simulink model "etherCATmdl"  (R2022a)
settings: Solver=FixedStepDiscrete  StartTime=0.0  StopTime=inf  FixedStep=0.001  RelTol=1e-3
PreLoadFcn:
  | Ts_IO133 = 0.001;
  | Ts_IO750 = 0.001;
InitFcn:
  | Ts_IO133 = 0.001
StopFcn:
  | if isfile(['sdi_view_',bdroot,'.mldatx'])
  |  Simulink.sdi.clearPreferences();
  |  Simulink.sdi.view();
  |  pause(3);
  |  Simulink.sdi.loadView(['sdi_view_',bdroot,]);
  | end
undefined symbols (not defined in the file or in its folder): AUS0, AUS1, C, CAN, FD, padding, Statuswort, Steuerwort
libraries: speedgoatlib_IO750 x12, speedgoatlib_IO602 x9, slrealtimeutilitieslib x8, slrealtimeloglib x6, speedgoatlib_IO133 x5, canfdmsglib x4, canmsglib x4, etargetslib x2, slrealtimeptplib x2, speedgoatlib_interrupt x1, simulink x1
settings Model: SimulationMode=external  ExtModeEnableFloating=off  Creator=sandro.reichenbach  LastModifiedBy=muhammet.cingoez
settings SolverCC: ConcurrentTasks=on  PositivePriorityOrder=on  AutoInsertRateTranBlk=on
settings DataIOCC: LimitDataPoints=on  SaveFormat=StructureWithTime
settings OptimizationCC: BlockReduction=off  OptimizeBlockIOStorage=off
settings DebuggingCC: TasksWithSamePriorityMsg=none
settings HardwareCC: ProdBitPerLong=64  ProdLongLongMode=on  ProdHWDeviceType=Intel->x86-64 (Linux 64)
settings RTWCC: Description=Simulink Real-Time  SystemTargetFile=slrealtime.tlc  TemplateMakefile=slrealtime_default_tmf  PostCodeGenCommand=sg.model.build.makeCfg(bdroot, buildInfo);  RTWVerbose=off  Toolchain=Simulink Real-Time Toolchain  BuildConfiguration=Faster Runs  CodeExecutionProfiling=on  TargetLang=C++  DLArmComputeVersion=19.05

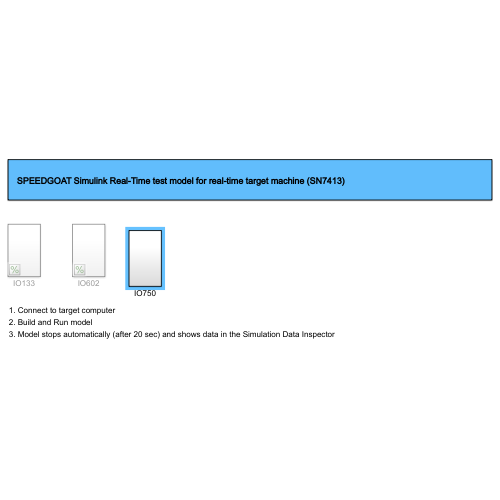
[thumbnail: Simulink's stored preview of the top-level diagram]
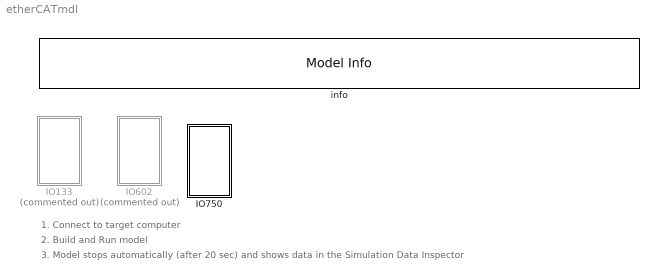
== system etherCATmdl ==
  note: 1. Connect to target computer
  note: 2. Build and Run model
  note: 3. Model stops automatically (after 20 sec) and shows data in the Simulation Data Inspector
  IO133 : Subsystem  Commented=on
  IO602 : Subsystem  Commented=on
  IO750 : Subsystem
  info : simulink/Model-Wide Utilities/Model Info  Frame=on  DisplayStringWithTags=SPEEDGOAT Simulink Real-Time test model for real-time target machine (SN7413)  HorizontalTextAlignment=Left  LeftAlignmentValue=0.02

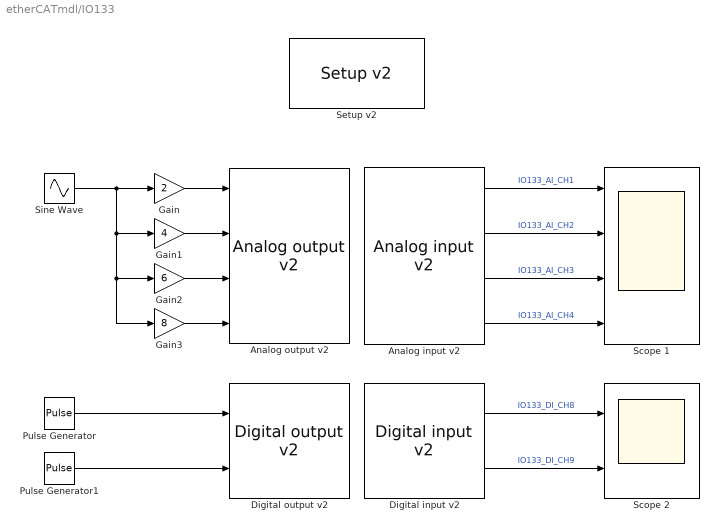
== system etherCATmdl/IO133 ==
  "Analog input v2 " : speedgoatlib_IO133/Analog input v2   parModuleId=1  parSampleTime=Ts_IO133  parPciSlot=-1  parAdcChannels=[1 2 3 4]  parAdcVoltageRange=[2 2]  parAdcOversamplRate=[1 1]  parAdcContSampling=0  parAdcDmaEnable=0  parAdcActiveDmaDevices=[1 1]  parAdcFrameSize=100
      settings: SourceProductName=Simulink Real-Time: Speedgoat I/O Driver Library
  "Analog output v2 " : speedgoatlib_IO133/Analog output v2   parModuleId=1  parSampleTime=Ts_IO133  parPciSlot=-1  parDacChannels=[1 2 3 4]  parDacVoltageRange=[4 4 6 6 5 5 5 5]  parDacInitValues=[0 0 0 0]  parDacReset=[1 1 1 1]  parDacSyncOut=1  parDacDmaEnable=0  parDacActiveDmaDevices=[1 1]  parDacDmaLatency=2  parDacFrameSize=100
      settings: SourceProductName=Simulink Real-Time: Speedgoat I/O Driver Library
  "Digital input v2 " : speedgoatlib_IO133/Digital input v2   parModuleId=1  parSampleTime=Ts_IO133  parPciSlot=-1  parDiChannels=[8 9]
      settings: SourceProductName=Simulink Real-Time: Speedgoat I/O Driver Library
  "Digital output v2 " : speedgoatlib_IO133/Digital output v2   parModuleId=1  parSampleTime=Ts_IO133  parPciSlot=-1  parDoChannels=[1 2]  parDoInitValues=[0 0]  parDoReset=[1 1]
      settings: SourceProductName=Simulink Real-Time: Speedgoat I/O Driver Library
  Gain : Gain  Gain=2
  Gain1 : Gain  Gain=4
  Gain2 : Gain  Gain=6
  Gain3 : Gain  Gain=8
  Pulse Generator : DiscretePulseGenerator  Period=20  PulseWidth=5  SampleTime=-1
  Pulse Generator1 : DiscretePulseGenerator  Period=20  PulseWidth=10  SampleTime=-1
  Scope 1 : Scope  NumInputPorts=4
  Scope 2 : Scope  NumInputPorts=2
  "Setup v2 " : speedgoatlib_IO133/Setup v2   parPciSlot=-1  parModuleId=1  parInterModuleSync=None  parConvClockBaseRate=20MHz  parConvClock1Divider=20000  parConvClock2Divider=20000  parFrameTriggerEnable=off  parFrameTriggerDivider=10  parConvClock1BaseRate=1  parConvClock2BaseRate=1  parFrameTriggerClock=1  parAdcChannels=1:4  parAdcRange1=+-10V  parAdcRange2=+-10V  parAdcVoltageRange=[2 2]  parAdcOversampling1=None  parAdcOversampling2=None  parAdcOversamplRate=[1 1]  parAdcAutoCorrection=on  parAdcContSampling=off  parAdcDmaEnable=off  parAdcDmaClock=Clock 1  parAdcFrameSize_=100  parAdcSampleTime_=-1  parAdcActiveDmaDevices=[1 1]  parAdcFrameTriggerEnable=0  parAdcFrameSize=100  parAdcSampleTime=0.1  parDacChannels=1:4  parDacInitValues=0  parDacReset=1  parDacRange1=+-5V  parDacRange2=+-5V  parDacRange3=+-10.8V  parDacRange4=+-10.8V  parDacRange5=+-10V  parDacRange6=+-10V  parDacRange7=+-10V  parDacRange8=+-10V  parDacVoltageRange=[4 4 6 6 5 5 5 5]  parDacAutoCorrection=on  parDacSyncOut=on  parDacDmaEnable=off  parDacDmaLatency=Until next frame  parDacDmaClock=Clock 1  parDacFrameSize_=100  parDacSampleTime_=-1  parDacActiveDmaDevices=[1 1]  parDacFrameTriggerEnable=0  parDacFrameSize=100  parDacSampleTime=0.1  parDoChannels=1:2  parDoInitValues=0  parDoReset=1  parDiChannels=8:9  parDiDebounceEnable=off  parDiDebounceTime=0  parDiDebounceValue=0  parDioPullRefFront=Pull-up 3.3V  parDioPullRefRear=Floating
      settings: SourceProductName=Simulink Real-Time: Speedgoat I/O Driver Library
  Sine Wave : Sin  Frequency=50  SampleTime=0
  wires:
  Pulse Generator/1 -> "Digital output v2 "/1
  Gain1/1 -> "Analog output v2 "/2
  Gain/1 -> "Analog output v2 "/1
  Gain3/1 -> "Analog output v2 "/4
  Gain2/1 -> "Analog output v2 "/3
  Sine Wave/1 -> Gain/1, Gain1/1, Gain2/1, Gain3/1
  Pulse Generator1/1 -> "Digital output v2 "/2
  "Analog input v2 "/1 -> Scope 1/1  "IO133_AI_CH1"
  "Analog input v2 "/2 -> Scope 1/2  "IO133_AI_CH2"
  "Analog input v2 "/3 -> Scope 1/3  "IO133_AI_CH3"
  "Analog input v2 "/4 -> Scope 1/4  "IO133_AI_CH4"
  "Digital input v2 "/1 -> Scope 2/1  "IO133_DI_CH8"
  "Digital input v2 "/2 -> Scope 2/2  "IO133_DI_CH9"

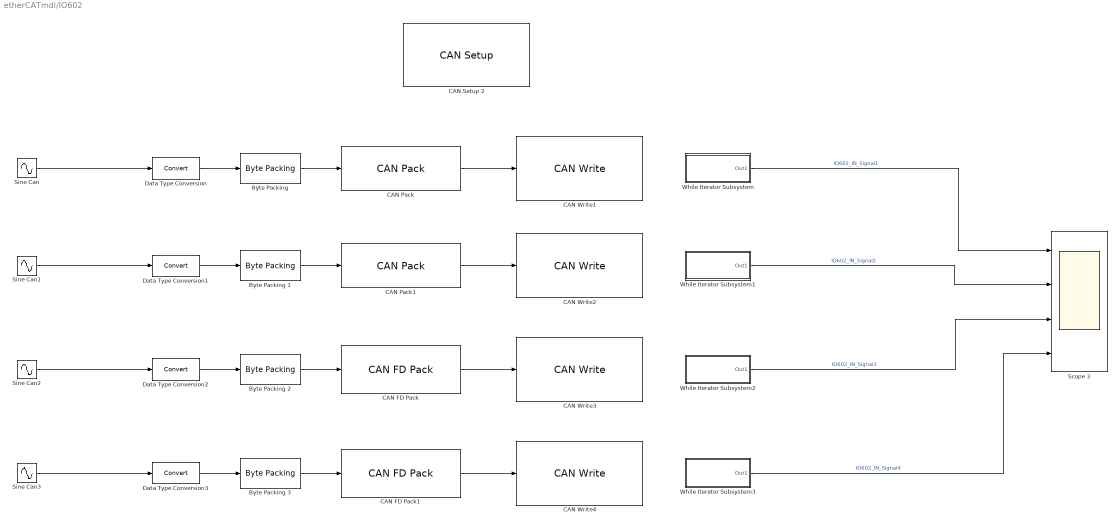
== system etherCATmdl/IO602 ==
  Byte Packing {,1..3} (4 alike) : slrealtimeutilitieslib/Byte Packing  MaskPackedDataType=uint8  MaskUnpackedDataTypes={'single'}  MaskAlignment=1
  CAN FD Pack : canfdmsglib/CAN FD Pack  MsgList=(none)  MsgName=Msg  ProtocolMode=CAN FD  MsgIDType=Standard (11-bit identifier)  MsgIdentifier=102  MsgLength=4  Remote=off  BRSSwitch=off  ApplyMinMax=off  SignalInfo={}
      settings: SourceProductBaseCode=XP,ME,VN  DataFormat=raw data
  CAN FD Pack1 : canfdmsglib/CAN FD Pack  MsgList=(none)  MsgName=Msg  ProtocolMode=CAN FD  MsgIDType=Standard (11-bit identifier)  MsgIdentifier=103  MsgLength=4  Remote=off  BRSSwitch=off  ApplyMinMax=off  SignalInfo={}
      settings: SourceProductBaseCode=XP,ME,VN  DataFormat=raw data
  CAN Pack : canmsglib/CAN Pack  MsgList=(none)  MsgName=CAN Msg  MsgIDType=Standard (11-bit identifier)  MsgIdentifier=100  MsgLength=4  Remote=off  ApplyMinMax=off  BusOutput=off  SignalInfo={}
      settings: SourceProductBaseCode=XP,ME,VN  DataFormat=raw data
  CAN Pack1 : canmsglib/CAN Pack  MsgList=(none)  MsgName=CAN Msg  MsgIDType=Standard (11-bit identifier)  MsgIdentifier=101  MsgLength=4  Remote=off  ApplyMinMax=off  BusOutput=off  SignalInfo={}
      settings: SourceProductBaseCode=XP,ME,VN  DataFormat=raw data
  CAN Setup 2 : speedgoatlib_IO602/Legacy/CAN Setup   moduletype=IO602  id=1  pciSlot=-1  chn1=CAN (HS)  chn2=CAN (HS)  chn3=CAN-FD  chn4=CAN-FD  initStruct=[]  termStruct=[]  ArbitrationbdrChn1=1.0 MBaud  ArbitrationManbdrChn1=[2,8,31,8]  FdbdrChn1=5.0 MBaud  FdManbdrChn1=[2,2,5,2]  ArbitrationbdrChn2=1.0 MBaud  ArbitrationManbdrChn2=[2,8,31,8]  FdbdrChn2=5.0 MBaud  FdManbdrChn2=[2,2,5,2]  ArbitrationbdrChn3=1.0 MBaud  ArbitrationManbdrChn3=[2,8,31,8]  FdbdrChn3=5.0 MBaud  FdManbdrChn3=[2,2,5,2]  ArbitrationbdrChn4=1.0 MBaud  ArbitrationManbdrChn4=[2,8,31,8]  FdbdrChn4=5.0 MBaud  FdManbdrChn4=[2,2,5,2]  moduleInitValues=[602 1 -1 -1]
      settings: SourceProductName=Simulink Real-Time: Speedgoat I/O Blockset
  CAN Write1 : speedgoatlib_IO602/Legacy/CAN Write  id=1  ts=-1  channel=1  messageType=CAN  BusInput=off  enableStatusPort=off  canType=CAN (HS)  initValues=[602 1 -1 0 1 1 0 0]
      settings: SourceProductName=Simulink Real-Time: Speedgoat I/O Blockset
  CAN Write2 : speedgoatlib_IO602/Legacy/CAN Write  id=1  ts=-1  channel=2  messageType=CAN  BusInput=off  enableStatusPort=off  canType=CAN (HS)  initValues=[602 1 -1 1 1 1 0 0]
      settings: SourceProductName=Simulink Real-Time: Speedgoat I/O Blockset
  CAN Write3 : speedgoatlib_IO602/Legacy/CAN Write  id=1  ts=-1  channel=3  messageType=CAN  BusInput=off  enableStatusPort=off  canType=CAN-FD  initValues=[602 1 -1 2 1 2 0 0]
      settings: SourceProductName=Simulink Real-Time: Speedgoat I/O Blockset
  CAN Write4 : speedgoatlib_IO602/Legacy/CAN Write  id=1  ts=-1  channel=4  messageType=CAN  BusInput=off  enableStatusPort=off  canType=CAN-FD  initValues=[602 1 -1 3 1 2 0 0]
      settings: SourceProductName=Simulink Real-Time: Speedgoat I/O Blockset
  Data Type Conversion{,1..3} (4 alike) : DataTypeConversion  SaturateOnIntegerOverflow=off  RndMeth=Floor
  Scope 3 : Scope  NumInputPorts=4
  Sine Can : Sin  Amplitude=50  Frequency=10*2*pi  SampleTime=0.005
  Sine Can1 : Sin  Amplitude=20  Frequency=10*2*pi  SampleTime=0.005
  Sine Can2 : Sin  Amplitude=30  Frequency=10*2*pi  SampleTime=0.005
  Sine Can3 : Sin  Amplitude=40  Frequency=10*2*pi  SampleTime=0.005
  While Iterator Subsystem : Subsystem  TreatAsAtomicUnit=on
  While Iterator Subsystem1 : Subsystem  TreatAsAtomicUnit=on
  While Iterator Subsystem2 : Subsystem  TreatAsAtomicUnit=on
  While Iterator Subsystem3 : Subsystem  TreatAsAtomicUnit=on
  wires:
  While Iterator Subsystem/1(Out1) -> Scope 3/1  "IO602_IN_Signal1"
  Data Type Conversion/1 -> "Byte Packing "/1
  Sine Can/1 -> Data Type Conversion/1
  CAN Pack/1 -> CAN Write1/1
  "Byte Packing "/1 -> CAN Pack/1
  Byte Packing 1/1 -> CAN Pack1/1
  CAN Pack1/1 -> CAN Write2/1
  Sine Can1/1 -> Data Type Conversion1/1
  Data Type Conversion1/1 -> Byte Packing 1/1
  While Iterator Subsystem1/1(Out1) -> Scope 3/2  "IO602_IN_Signal2"
  While Iterator Subsystem3/1(Out1) -> Scope 3/4  "IO602_IN_Signal4"
  Data Type Conversion3/1 -> Byte Packing 3/1
  Sine Can3/1 -> Data Type Conversion3/1
  CAN FD Pack1/1 -> CAN Write4/1
  Byte Packing 3/1 -> CAN FD Pack1/1
  Byte Packing 2/1 -> CAN FD Pack/1
  CAN FD Pack/1 -> CAN Write3/1
  Sine Can2/1 -> Data Type Conversion2/1
  Data Type Conversion2/1 -> Byte Packing 2/1
  While Iterator Subsystem2/1(Out1) -> Scope 3/3  "IO602_IN_Signal3"

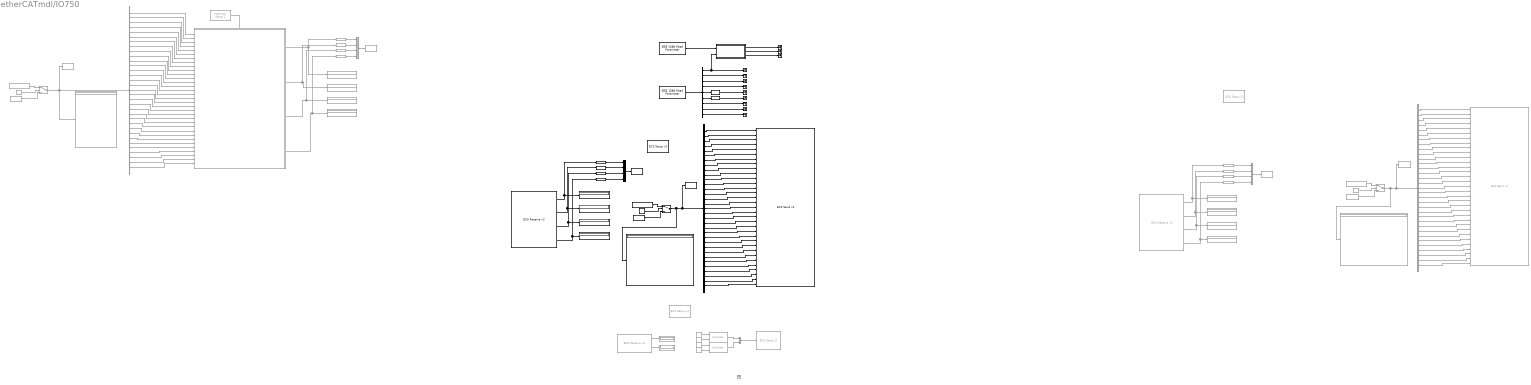
== system etherCATmdl/IO750 ==
  note: Update System Time
      | To sync the system time of the target use the following command:
      | >> speedgoat.setTargetTime
      |
      | for more information please refer to the MathWorks documentation:
      | web(fullfile(docroot, 'slrealtime/api/slrealtime.target.ptpd.html'))
  Bias : Bias  Bias=1  SaturateOnIntegerOverflow=off
  Bias1 : Bias  Bias=1900  SaturateOnIntegerOverflow=off
  Byte Pack1 : etargetslib/Byte Pack  Commented=on  datatypes={'uint32','single'}  byteAlign=1
  Byte Pack2 : etargetslib/Byte Pack  Commented=on  datatypes={'uint32','single'}  byteAlign=1
  Constant : Constant  Value=0  SampleTime=-1
  Constant1 : Constant  Commented=on  Value=12  OutDataTypeStr=uint32
  Constant10 : Constant  Commented=on
  Constant11 : Constant  Commented=on  Value=double(randi(250,1,33))
  Constant12 : Constant  Commented=on  Value=zeros(1,33)  OutDataTypeStr=double
  Constant2 : Constant  Commented=on  Value=39  OutDataTypeStr=single
  Constant3 : Constant  Commented=on  Value=26  OutDataTypeStr=uint32
  Constant4 : Constant  Commented=on  Value=11  OutDataTypeStr=single
  Constant5 : Constant  Value=double(randi(250,1,33))  SampleTime=-1
  Constant6 : Constant  Value=zeros(1,33)  OutDataTypeStr=double  SampleTime=-1
  Constant7 : Constant  Commented=on  Value=0
  Constant8 : Constant  Commented=on  Value=double(randi(250,1,33))
  Constant9 : Constant  Commented=on  Value=zeros(1,33)  OutDataTypeStr=double
  Data Type Conversion{1..4} (4 alike) : DataTypeConversion  SaturateOnIntegerOverflow=off  RndMeth=Floor
  Data Type Conversion{5..12} (8 alike) : DataTypeConversion  Commented=on  SaturateOnIntegerOverflow=off  RndMeth=Floor
  Demux : Demux  Outputs=33
  Demux1 : Demux  Outputs=9
  Demux2 : Demux  Commented=on  Outputs=33
  Demux3 : Demux  Commented=on  Outputs=33
  Display{,1,7..16} (12 alike) : Display  Commented=on
  Display{2..6} (5 alike) : Display
  "ECS Receive v2 " : speedgoatlib_IO750/ECS Receive v2   id=1  portType=Separate signals  sampleTime=Ts_IO750  pdoTable={ 'Rx PDO1', 'myvar1', 'uint8'; 'Rx PDO1', 'myvar2', 'single'; 'Rx PDO2', 'myvar1', 'int16'; 'Rx PDO3', 'myvar1', 'double' }
      settings: SourceProductName=Simulink Real-Time: Speedgoat I/O Blockset
  ECS Receive v2 1 : speedgoatlib_IO750/ECS Receive v2   Commented=on  id=1  portType=Separate signals  sampleTime=Ts_IO750  pdoTable={ 'Rx', 'ControlSpeed', 'uint32'; 'Rx', 'ControlWord', 'single' }
      settings: SourceProductName=Simulink Real-Time: Speedgoat I/O Blockset
  ECS Receive v2 2 : speedgoatlib_IO750/ECS Receive v2   Commented=on  id=1  portType=Separate signals  sampleTime=Ts_IO750  pdoTable={ 'Rx PDO1', 'myvar1', 'uint8'; 'Rx PDO1', 'myvar2', 'single'; 'Rx PDO2', 'myvar1', 'int16'; 'Rx PDO3', 'myvar1', 'double' }
      settings: SourceProductName=Simulink Real-Time: Speedgoat I/O Blockset
  "ECS Send v2 " : speedgoatlib_IO750/ECS Send v2   id=1  portType=Separate signals  sampleTime=-1  pdoTable={ 'Tx PDO1', 'myvar1', 'double'; 'Tx PDO2', 'myvar2', 'double'; 'Tx PDO3', 'myvar3', 'double'; 'Tx PDO4', 'myvar4', 'double'; 'Tx PDO5', 'myvar5', 'double'; 'Tx PDO6', 'myvar6', 'double'; 'Tx PDO7', 'myvar7', 'double'; 'Tx PDO8', 'myvar8', 'double'; 'Tx PDO9', 'myvar9', 'double'; 'Tx PDO10', 'myvar10', 'double'; 'Tx PDO11', 'myvar11', 'double'; 'Tx PDO12', 'myvar12', 'double'; 'Tx PDO13', 'myvar13', 'double'; 'Tx PDO14', 'myvar14', 'double'; 'Tx PDO15', 'myvar15', 'double'; 'Tx PDO16', 'myvar16', 'double'; 'Tx PDO17', 'myvar17', 'double'; 'Tx PDO18', 'myvar18', 'double'; 'Tx PDO19', 'myvar19', 'double'; 'Tx PDO20', 'myvar20', 'double'; 'Tx PDO21', 'myvar21', 'double'; 'Tx PDO22', 'myvar22', 'double'; 'Tx PDO23', 'myvar23', 'double'; 'Tx PDO24', 'myvar24', 'double'; 'Tx PDO25', 'myvar25', 'double'; 'Tx PDO26', 'myvar26', 'double'; 'Tx PDO27', 'myvar27', 'double'; 'Tx PDO28', 'myvar28', 'double'; 'Tx PDO29', 'myvar29', 'double'; 'Tx PDO30', 'myvar30', 'double'; 'Tx PDO31', 'myvar31', 'double'; 'Tx PDO32', 'myvar32', 'double'; 'Tx PDO32', 'myvar33', 'double' }
      settings: SourceProductName=Simulink Real-Time: Speedgoat I/O Blockset
  ECS Send v2 1 : speedgoatlib_IO750/ECS Send v2   Commented=on  id=1  portType=Byte vector  sampleTime=-1  pdoTable={ 'Tx', 'ActualSpeed', 'uint32'; 'Tx', 'StatusWord', 'single'; 'Tx', 'var_3', 'uint32'; 'Tx', 'var_4', 'single' }
      settings: SourceProductName=Simulink Real-Time: Speedgoat I/O Blockset
  ECS Send v2 2 : speedgoatlib_IO750/ECS Send v2   Commented=on  id=1  portType=Separate signals  sampleTime=-1  pdoTable={ 'Tx PDO1', 'myvar1', 'double'; 'Tx PDO2', 'myvar2', 'double'; 'Tx PDO3', 'myvar3', 'double'; 'Tx PDO4', 'myvar4', 'double'; 'Tx PDO5', 'myvar5', 'double'; 'Tx PDO6', 'myvar6', 'double'; 'Tx PDO7', 'myvar7', 'double'; 'Tx PDO8', 'myvar8', 'double'; 'Tx PDO9', 'myvar9', 'double'; 'Tx PDO10', 'myvar10', 'double'; 'Tx PDO11', 'myvar11', 'double'; 'Tx PDO12', 'myvar12', 'double'; 'Tx PDO13', 'myvar13', 'double'; 'Tx PDO14', 'myvar14', 'double'; 'Tx PDO15', 'myvar15', 'double'; 'Tx PDO16', 'myvar16', 'double'; 'Tx PDO17', 'myvar17', 'double'; 'Tx PDO18', 'myvar18', 'double'; 'Tx PDO19', 'myvar19', 'double'; 'Tx PDO20', 'myvar20', 'double'; 'Tx PDO21', 'myvar21', 'double'; 'Tx PDO22', 'myvar22', 'double'; 'Tx PDO23', 'myvar23', 'double'; 'Tx PDO24', 'myvar24', 'double'; 'Tx PDO25', 'myvar25', 'double'; 'Tx PDO26', 'myvar26', 'double'; 'Tx PDO27', 'myvar27', 'double'; 'Tx PDO28', 'myvar28', 'double'; 'Tx PDO29', 'myvar29', 'double'; 'Tx PDO30', 'myvar30', 'double'; 'Tx PDO31', 'myvar31', 'double'; 'Tx PDO32', 'myvar32', 'double'; 'Tx PDO32', 'myvar33', 'double' }
      settings: SourceProductName=Simulink Real-Time: Speedgoat I/O Blockset
  "ECS Setup v2 " : speedgoatlib_IO750/ECS Setup v2   Commented=on  id=1  drvLetter=C:  configurationMode=Warmstart  busSlot=-1  busStartup=Automatic  dcSync=on  vendorName='Speedgoat'  groupName='Automation'  typeName='IO750'  vendorID=hex2dec('00000001')  productCode=hex2dec('00000002')  revisionNo=hex2dec('00000003')  serialNo=hex2dec('00000004')  stationAlias=0  deviceIdent=0  rxPdoMapping={'Rx1','myvar1','double';'Rx2','myvar2','double';'Rx3','myvar3','double';'Rx4','myvar4','double';'Rx5','myvar5','double';'Rx6','myvar6','double';'Rx7','myvar7','double';'Rx8','myvar8','double';'Rx9','myvar9','double';'Rx10','myvar10','double';'Rx11','myvar11','double';'Rx12','myvar12','double';'Rx13','myvar13','double';'Rx14','myvar14','double';'Rx15','myvar15','double';'Rx16','myvar16','double';'Rx17','myvar17','double';'Rx18','myvar18','double';'Rx19','myvar19','double';'Rx20','myvar20','double';'Rx21','myvar21','double';'Rx22','myvar22','double';'Rx23','myvar23','double';'Rx24','myvar24','double';'Rx25','myvar25','double';'Rx26','myvar26','double';'Rx27','myvar27','double';'Rx28','myvar28','double';'Rx29','myvar29','double';'Rx30','myvar30','double';'Rx31','myvar31','double';'Rx32','myvar32','double';'Rx33','myvar33','double';'Rx34','myvar34','double';'Rx35','myvar35','double';'Rx36','myvar36','double';'Rx37','myvar37','double';'Rx38','myvar38','double';'Rx39','myvar39','double';'Rx40','myvar40','double';'Rx41','myvar41','double';'Rx42','myvar42','double';'Rx43','myvar43','double';'Rx44','myvar44','double';'Rx45','myvar45','double';'Rx46','myvar46','double';'Rx47','myvar47','double';'Rx48','myvar48','double';'Rx49','myvar49','double';'Rx50','myvar50','double';'Rx51','myvar51','double';'Rx52','myvar52','double';'Rx53','myvar53','double';'Rx54','myvar54','double';'Rx55','myvar55','double';'Rx56','myvar56','double';'Rx57','myvar57','double';'Rx58','myvar58','double';'Rx59','myvar59','double';'Rx60','myvar60','double';'Rx61','myvar61','double';'Rx62','myvar62','double';}  rxPdoCfg=0  rxPdoNames=,Steuerwort,Steuerwort,Statuswort  rxVarNames=,AUS0,padding,AUS1  txPdoMapping={'PDO1','myvar1','single';'PDO2','myvar2','single';'PDO3','myvar3','single';'PDO4','myvar4','single';'PDO5','myvar5','single';'PDO6','myvar6','single';'PDO7','myvar7','single';'PDO8','myvar8','single';'PDO9','myvar9','single';'PDO10','myvar10','single';'PDO11','myvar11','single';'PDO12','myvar12','single';'PDO13','myvar13','single';'PDO14','myvar14','single';'PDO15','myvar15','single';'PDO16','myvar16','single';'PDO17','myvar17','single';'PDO18','myvar18','single';'PDO19','myvar19','single';'PDO20','myvar20','single';'PDO21','myvar21','single';'PDO22','myvar22','single';'PDO23','myvar23','single';'PDO24','myvar24','single';'PDO25','myvar25','single';'PDO26','myvar26','single';'PDO27','myvar27','single';'PDO28','myvar28','single';'PDO29','myvar29','single';'PDO30','myvar30','single';'PDO31','myvar31','single';'PDO32','myvar32','single';'PDO33','myvar33','single';'PDO34','myvar34','single';'PDO35','myvar35','single';'PDO36','myvar36','single';'PDO37','myvar37','single';'PDO38','myvar38','single';'PDO39','myvar39','single';'PDO40','myvar40','single';'PDO41','myvar41','single';'PDO42','myvar42','single';'PDO43','myvar43','single';'PDO44','myvar44','single';'PDO45','myvar45','single';'PDO46','myvar46','single';'PDO47','myvar47','single';'PDO48','myvar48','single';'PDO49','myvar49','single';'PDO50','myvar50','single';'PDO51','myvar51','single';'PDO52','myvar52','single';'PDO53','myvar53','single';'PDO54','myvar54','single';'PDO55','myvar55','single';'PDO56','myvar56','single';'PDO57','myvar57','single';'PDO58','myvar58','single';'PDO59','myvar59','single';'PDO60','myvar60','single';'PDO61','myvar61','single';'PDO62','myvar62','single';'PDO63','myvar63','single';'PDO64','myvar64','single';'PDO65','myvar65','single';'PDO66','myvar66','single';'PDO67','myvar67','single';'PDO68','myvar68','single';'PDO69','myvar69','single';'PDO70','myvar70','single';}  txPdoCfg=0  txPdoNames=0  txVarNames=0  sdoMapping={}  sdoCfg=0  sdoNames=0  qtyMods=[1,0,0]  moduleType=IO750  protocol=IO750  firmware=EtherCAT Slave
      settings: SourceProductName=Simulink Real-Time: Speedgoat I/O Blockset
  ECS Setup v2 1 : speedgoatlib_IO750/ECS Setup v2   Commented=on  id=1  drvLetter=C:  configurationMode=Warmstart  busSlot=-1  busStartup=Automatic  dcSync=off  vendorName='Speedgoat'  groupName='Automation'  typeName='IO750'  vendorID=hex2dec('00000001')  productCode=hex2dec('00000002')  revisionNo=hex2dec('00000003')  serialNo=hex2dec('00000004')  stationAlias=0  deviceIdent=0  rxPdoMapping={ 'Rx', 'ControlSpeed', 'uint32'; 'Rx', 'ControlWord', 'single' }  rxPdoCfg=0  rxPdoNames=,Steuerwort,Steuerwort,Statuswort  rxVarNames=,AUS0,padding,AUS1  txPdoMapping={ 'Tx', 'ActualSpeed', 'uint32'; 'Tx', 'StatusWord', 'single'; 'Tx', 'var_3', 'uint32'; 'Tx', 'var_4', 'single' }  txPdoCfg=0  txPdoNames=0  txVarNames=0  sdoMapping={}  sdoCfg=0  sdoNames=0  qtyMods=[1,0,0]  moduleType=IO750  protocol=IO750  firmware=EtherCAT Slave
      settings: SourceProductName=Simulink Real-Time: Speedgoat I/O Blockset
  ECS Setup v2 2 : speedgoatlib_IO750/ECS Setup v2   id=1  drvLetter=C:  configurationMode=Warmstart  busSlot=-1  busStartup=Automatic  dcSync=off  vendorName='Speedgoat'  groupName='Automation'  typeName='IO750'  vendorID=hex2dec('00000001')  productCode=hex2dec('00000002')  revisionNo=hex2dec('00000003')  serialNo=hex2dec('00000004')  stationAlias=0  deviceIdent=0  rxPdoMapping={ 'Rx PDO1', 'myvar1', 'uint8'; 'Rx PDO1', 'myvar2', 'single'; 'Rx PDO2', 'myvar1', 'int16'; 'Rx PDO3', 'myvar1', 'double' }  rxPdoCfg=0  rxPdoNames=,Steuerwort,Steuerwort,Statuswort  rxVarNames=,AUS0,padding,AUS1  txPdoMapping={ 'Tx PDO1', 'myvar1', 'double'; 'Tx PDO2', 'myvar2', 'double'; 'Tx PDO3', 'myvar3', 'double'; 'Tx PDO4', 'myvar4', 'double'; 'Tx PDO5', 'myvar5', 'double'; 'Tx PDO6', 'myvar6', 'double'; 'Tx PDO7', 'myvar7', 'double'; 'Tx PDO8', 'myvar8', 'double'; 'Tx PDO9', 'myvar9', 'double'; 'Tx PDO10', 'myvar10', 'double'; 'Tx PDO11', 'myvar11', 'double'; 'Tx PDO12', 'myvar12', 'double'; 'Tx PDO13', 'myvar13', 'double'; 'Tx PDO14', 'myvar14', 'double'; 'Tx PDO15', 'myvar15', 'double'; 'Tx PDO16', 'myvar16', 'double'; 'Tx PDO17', 'myvar17', 'double'; 'Tx PDO18', 'myvar18', 'double'; 'Tx PDO19', 'myvar19', 'double'; 'Tx PDO20', 'myvar20', 'double'; 'Tx PDO21', 'myvar21', 'double'; 'Tx PDO22', 'myvar22', 'double'; 'Tx PDO23', 'myvar23', 'double'; 'Tx PDO24', 'myvar24', 'double'; 'Tx PDO25', 'myvar25', 'double'; 'Tx PDO26', 'myvar26', 'double'; 'Tx PDO27', 'myvar27', 'double'; 'Tx PDO28', 'myvar28', 'double'; 'Tx PDO29', 'myvar29', 'double'; 'Tx PDO30', 'myvar30', 'double'; 'Tx PDO31', 'myvar31', 'double'; 'Tx PDO32', 'myvar32', 'double'; 'Tx PDO32', 'myvar33', 'double' }  txPdoCfg=0  txPdoNames=0  txVarNames=0  sdoMapping={}  sdoCfg=0  sdoNames=0  qtyMods=[1,0,0]  moduleType=IO750  protocol=IO750  firmware=EtherCAT Slave
      settings: SourceProductName=Simulink Real-Time: Speedgoat I/O Blockset
  File Log : slrealtimeloglib/File Log  decimation=1  inputProcessing=Elements as channels (sample based)
      settings: SourceProductBaseCode=XP
  File Log1 : slrealtimeloglib/File Log  decimation=1  inputProcessing=Elements as channels (sample based)
      settings: SourceProductBaseCode=XP
  File Log{2..5} (4 alike) : slrealtimeloglib/File Log  Commented=on  decimation=1  inputProcessing=Elements as channels (sample based)
      settings: SourceProductBaseCode=XP
  Function-Call Subsystem : Subsystem  Commented=on  TreatAsAtomicUnit=on
  IEEE 1588 Read Parameter : slrealtimeptplib/IEEE 1588 Read Parameter  Priority=1  ID=1  param=1. System time (nanosecond)  sample_time=-1
      settings: SourceProductBaseCode=XP
  IEEE 1588 Read Parameter1 : slrealtimeptplib/IEEE 1588 Read Parameter  Priority=1  ID=1  param=2. Calendar time (time_t)  sample_time=-1
      settings: SourceProductBaseCode=XP
  Interrupt Setup 1 : speedgoatlib_interrupt/Interrupt Setup 1  Commented=on  parModuleTrigger=off  parPollingMode=off  parPriorityConf=High  parPriority=241  confStartFcn=IO75x_start_public  confStopFcn=IO75x_stop_public  confIsrFcn=IO75x_isr_public  confMapFcn=IO75x_map_public  confHookFile=io75x_int_hooks.c  confIrqNr=-1  confIsMdlTrig=off  confIsPolling=off  confPriority=254  confModID=16776961  confSelectedInt=Speedgoat IO75x interrupt  confSelectedId=1
  MATLAB Function : MATLAB Function  TreatAsAtomicUnit=on
  Mux : Mux  Commented=on  Inputs=2
  Mux1 : Mux
  Mux2 : Mux  Commented=on
  Mux3 : Mux  Commented=on
  Switch : Switch  Criteria=u2 > Threshold  SaturateOnIntegerOverflow=off  InputSameDT=off
  Switch1 : Switch  Commented=on  Criteria=u2 > Threshold  SaturateOnIntegerOverflow=off  InputSameDT=off
  Switch2 : Switch  Commented=on  Criteria=u2 > Threshold  SaturateOnIntegerOverflow=off  InputSameDT=off
  Terminator : Terminator  Commented=on
  Terminator{1..12} (12 alike) : Terminator
  wires:
  Constant3/1 -> Byte Pack1/1
  Constant4/1 -> Byte Pack1/2
  Mux/1 -> ECS Send v2 1/1
  Byte Pack1/1 -> Mux/1
  Constant2/1 -> Byte Pack2/2
  Constant1/1 -> Byte Pack2/1
  Byte Pack2/1 -> Mux/2
  Switch/1 -> Display2/1, File Log1/1, Demux/1  "SentPack2"
  "ECS Receive v2 "/2 -> Data Type Conversion2/1, Display4/1
  "ECS Receive v2 "/3 -> Data Type Conversion3/1, Display5/1
  "ECS Receive v2 "/4 -> Data Type Conversion4/1, Display6/1
  "ECS Receive v2 "/1 -> Data Type Conversion1/1, Display3/1
  Mux1/1 -> File Log/1
  Data Type Conversion1/1 -> Mux1/1
  Data Type Conversion2/1 -> Mux1/2
  Data Type Conversion3/1 -> Mux1/3
  Data Type Conversion4/1 -> Mux1/4
  Constant5/1 -> Switch/1  "SentPack2"
  Constant/1 -> Switch/2
  Constant6/1 -> Switch/3
  ECS Receive v2 1/1 -> Display/1
  ECS Receive v2 1/2 -> Display1/1
  Demux/1 -> "ECS Send v2 "/1
  Demux/2 -> "ECS Send v2 "/2
  Demux/3 -> "ECS Send v2 "/3
  Demux/4 -> "ECS Send v2 "/4
  Demux/5 -> "ECS Send v2 "/5
  Demux/6 -> "ECS Send v2 "/6
  Demux/7 -> "ECS Send v2 "/7
  Demux/8 -> "ECS Send v2 "/8
  Demux/9 -> "ECS Send v2 "/9
  Demux/10 -> "ECS Send v2 "/10
  Demux/11 -> "ECS Send v2 "/11
  Demux/12 -> "ECS Send v2 "/12
  Demux/13 -> "ECS Send v2 "/13
  Demux/14 -> "ECS Send v2 "/14
  Demux/15 -> "ECS Send v2 "/15
  Demux/16 -> "ECS Send v2 "/16
  Demux/17 -> "ECS Send v2 "/17
  Demux/18 -> "ECS Send v2 "/18
  Demux/19 -> "ECS Send v2 "/19
  Demux/20 -> "ECS Send v2 "/20
  Demux/21 -> "ECS Send v2 "/21
  Demux/22 -> "ECS Send v2 "/22
  Demux/23 -> "ECS Send v2 "/23
  Demux/24 -> "ECS Send v2 "/24
  Demux/25 -> "ECS Send v2 "/25
  Demux/26 -> "ECS Send v2 "/26
  Demux/27 -> "ECS Send v2 "/27
  Demux/28 -> "ECS Send v2 "/28
  Demux/29 -> "ECS Send v2 "/29
  Demux/30 -> "ECS Send v2 "/30
  Demux/31 -> "ECS Send v2 "/31
  Demux/32 -> "ECS Send v2 "/32
  Demux/33 -> "ECS Send v2 "/33
  MATLAB Function/2(microseconds) -> Terminator11/1  "microseconds"
  Demux1/8 -> Terminator9/1
  Demux1/5 -> Bias/1
  Demux1/3 -> Terminator4/1  "hours"
  Demux1/9 -> Terminator12/1
  Demux1/4 -> Terminator5/1  "day"
  MATLAB Function/3(miliseconds) -> Terminator10/1  "milliseconds"
  IEEE 1588 Read Parameter/1 -> MATLAB Function/1(nanosecondsAbs)  "abs_nanoseconds"
  Bias/1 -> Terminator6/1  "month"
  IEEE 1588 Read Parameter1/1 -> Demux1/1  "cal_time"
  Demux1/1 -> MATLAB Function/2(secondsIn), Terminator2/1  "seconds"
  Bias1/1 -> Terminator7/1  "year"
  Demux1/2 -> Terminator3/1  "minutes"
  MATLAB Function/1(nanoseconds) -> Terminator1/1  "nanoseconds"
  Demux1/7 -> Terminator8/1
  Demux1/6 -> Bias1/1
  Demux2/33 -> ECS Send v2 2/33
  Demux2/32 -> ECS Send v2 2/32
  Demux2/31 -> ECS Send v2 2/31
  Demux2/30 -> ECS Send v2 2/30
  Demux2/29 -> ECS Send v2 2/29
  Demux2/28 -> ECS Send v2 2/28
  Demux2/27 -> ECS Send v2 2/27
  Demux2/26 -> ECS Send v2 2/26
  Demux2/25 -> ECS Send v2 2/25
  Demux2/24 -> ECS Send v2 2/24
  Demux2/23 -> ECS Send v2 2/23
  Demux2/22 -> ECS Send v2 2/22
  Demux2/21 -> ECS Send v2 2/21
  Demux2/20 -> ECS Send v2 2/20
  Demux2/19 -> ECS Send v2 2/19
  Demux2/18 -> ECS Send v2 2/18
  Demux2/17 -> ECS Send v2 2/17
  Demux2/16 -> ECS Send v2 2/16
  Demux2/15 -> ECS Send v2 2/15
  Demux2/14 -> ECS Send v2 2/14
  Demux2/13 -> ECS Send v2 2/13
  Demux2/12 -> ECS Send v2 2/12
  Demux2/11 -> ECS Send v2 2/11
  Demux2/10 -> ECS Send v2 2/10
  Demux2/9 -> ECS Send v2 2/9
  Demux2/8 -> ECS Send v2 2/8
  Demux2/7 -> ECS Send v2 2/7
  Demux2/6 -> ECS Send v2 2/6
  Demux2/5 -> ECS Send v2 2/5
  Demux2/4 -> ECS Send v2 2/4
  Demux2/3 -> ECS Send v2 2/3
  Demux2/2 -> ECS Send v2 2/2
  Demux2/1 -> ECS Send v2 2/1
  Constant9/1 -> Switch1/3
  Constant7/1 -> Switch1/2
  Constant8/1 -> Switch1/1  "SentPack2"
  Data Type Conversion8/1 -> Mux2/4
  Data Type Conversion7/1 -> Mux2/3
  Data Type Conversion6/1 -> Mux2/2
  Data Type Conversion5/1 -> Mux2/1
  Mux2/1 -> File Log2/1
  ECS Receive v2 2/1 -> Display8/1, Data Type Conversion5/1
  ECS Receive v2 2/4 -> Display11/1, Data Type Conversion8/1
  ECS Receive v2 2/3 -> Display10/1, Data Type Conversion7/1
  ECS Receive v2 2/2 -> Display9/1, Data Type Conversion6/1
  Switch1/1 -> Demux2/1, File Log3/1, Display7/1  "SentPack2"
  Constant12/1 -> Switch2/3
  Constant10/1 -> Switch2/2
  Constant11/1 -> Switch2/1  "SentPack2"
  Data Type Conversion12/1 -> Mux3/4
  Data Type Conversion11/1 -> Mux3/3
  Data Type Conversion10/1 -> Mux3/2
  Data Type Conversion9/1 -> Mux3/1
  Mux3/1 -> File Log4/1
  Switch2/1 -> Display12/1, Demux3/1, File Log5/1  "SentPack2"
  Interrupt Setup 1/1 -> Function-Call Subsystem/Trigger
  Demux3/28 -> Function-Call Subsystem/28(In28)
  Demux3/27 -> Function-Call Subsystem/27(In27)
  Demux3/29 -> Function-Call Subsystem/29(In29)
  Demux3/26 -> Function-Call Subsystem/26(In26)
  Demux3/30 -> Function-Call Subsystem/30(In30)
  Demux3/25 -> Function-Call Subsystem/25(In25)
  Demux3/31 -> Function-Call Subsystem/31(In31)
  Demux3/24 -> Function-Call Subsystem/24(In24)
  Demux3/32 -> Function-Call Subsystem/32(In32)
  Demux3/23 -> Function-Call Subsystem/23(In23)
  Demux3/33 -> Function-Call Subsystem/33(In33)
  Demux3/22 -> Function-Call Subsystem/22(In22)
  Demux3/21 -> Function-Call Subsystem/21(In21)
  Demux3/20 -> Function-Call Subsystem/20(In20)
  Demux3/19 -> Function-Call Subsystem/19(In19)
  Demux3/18 -> Function-Call Subsystem/18(In18)
  Demux3/17 -> Function-Call Subsystem/17(In17)
  Demux3/16 -> Function-Call Subsystem/16(In16)
  Demux3/15 -> Function-Call Subsystem/15(In15)
  Demux3/14 -> Function-Call Subsystem/14(In14)
  Demux3/13 -> Function-Call Subsystem/13(In13)
  Demux3/12 -> Function-Call Subsystem/12(In12)
  Demux3/11 -> Function-Call Subsystem/11(In11)
  Demux3/10 -> Function-Call Subsystem/10(In10)
  Demux3/9 -> Function-Call Subsystem/9(In9)
  Demux3/8 -> Function-Call Subsystem/8(In8)
  Demux3/7 -> Function-Call Subsystem/7(In7)
  Demux3/6 -> Function-Call Subsystem/6(In6)
  Demux3/5 -> Function-Call Subsystem/5(In5)
  Demux3/4 -> Function-Call Subsystem/4(In4)
  Demux3/3 -> Function-Call Subsystem/3(In3)
  Demux3/2 -> Function-Call Subsystem/2(In2)
  Demux3/1 -> Function-Call Subsystem/1(In1)
  Function-Call Subsystem/2(Out2) -> Data Type Conversion10/1, Display14/1
  Function-Call Subsystem/3(Out3) -> Data Type Conversion11/1, Display15/1
  Function-Call Subsystem/1(Out1) -> Data Type Conversion9/1, Display13/1
  Function-Call Subsystem/4(Out4) -> Data Type Conversion12/1, Display16/1

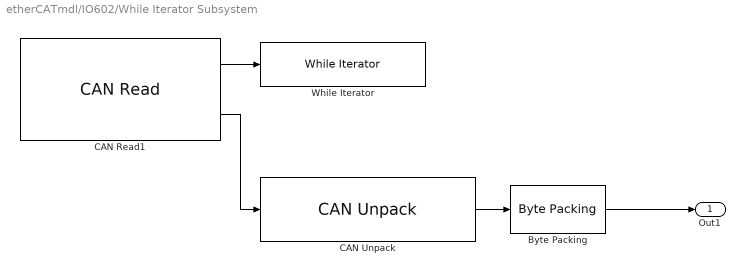
== system etherCATmdl/IO602/While Iterator Subsystem ==
  "Byte Packing " : slrealtimeutilitieslib/Byte Packing  MaskPackedDataType=single  MaskUnpackedDataTypes={'uint8'}  MaskAlignment=1
  CAN Read1 : speedgoatlib_IO602/Legacy/CAN Read  id=1  ts=-1  channel=1  messageType=CAN  canType=CAN (HS)  BusOutput=off  initValues=[602 1 -1 0 1 1 0]
      settings: SourceProductName=Simulink Real-Time: Speedgoat I/O Blockset
  CAN Unpack : canmsglib/CAN Unpack  MsgList=(none)  MsgName=CAN Msg  MsgIDType=Standard (11-bit identifier)  MsgIdentifier=101  MsgLength=4  SignalInfo={}  IDPort=off  TimestampPort=off  ErrorPort=off  RemotePort=off  LengthPort=off  StatusPort=off  ApplyMinMax=off
      settings: SourceProductBaseCode=XP,ME,VN  DataFormat=raw data
  While Iterator : WhileIterator  MaxIters=50  WhileBlockType=do-while
  Out1 : Outport
  wires:
  "Byte Packing "/1 -> Out1/1
  CAN Unpack/1 -> "Byte Packing "/1
  CAN Read1/2 -> CAN Unpack/1
  CAN Read1/1 -> While Iterator/1

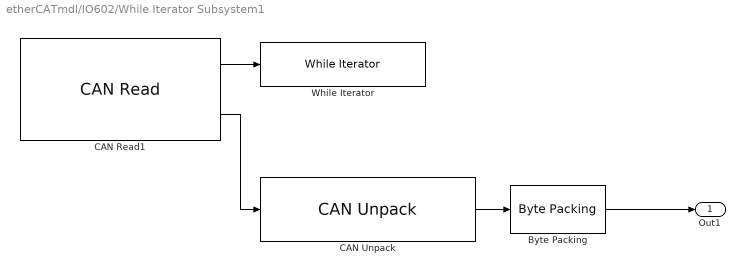
== system etherCATmdl/IO602/While Iterator Subsystem1 ==
  "Byte Packing " : slrealtimeutilitieslib/Byte Packing  MaskPackedDataType=single  MaskUnpackedDataTypes={'uint8'}  MaskAlignment=1
  CAN Read1 : speedgoatlib_IO602/Legacy/CAN Read  id=1  ts=-1  channel=2  messageType=CAN  canType=CAN (HS)  BusOutput=off  initValues=[602 1 -1 1 1 1 0]
      settings: SourceProductName=Simulink Real-Time: Speedgoat I/O Blockset
  CAN Unpack : canmsglib/CAN Unpack  MsgList=(none)  MsgName=CAN Msg  MsgIDType=Standard (11-bit identifier)  MsgIdentifier=100  MsgLength=4  SignalInfo={}  IDPort=off  TimestampPort=off  ErrorPort=off  RemotePort=off  LengthPort=off  StatusPort=off  ApplyMinMax=off
      settings: SourceProductBaseCode=XP,ME,VN  DataFormat=raw data
  While Iterator : WhileIterator  MaxIters=50  WhileBlockType=do-while
  Out1 : Outport
  wires:
  CAN Read1/1 -> While Iterator/1
  CAN Read1/2 -> CAN Unpack/1
  CAN Unpack/1 -> "Byte Packing "/1
  "Byte Packing "/1 -> Out1/1

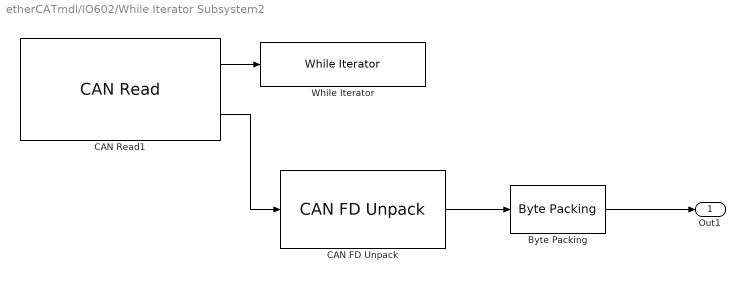
== system etherCATmdl/IO602/While Iterator Subsystem2 ==
  "Byte Packing " : slrealtimeutilitieslib/Byte Packing  MaskPackedDataType=single  MaskUnpackedDataTypes={'uint8'}  MaskAlignment=1
  CAN FD Unpack : canfdmsglib/CAN FD Unpack  MsgList=(none)  MsgName=Msg  ProtocolMode=CAN FD  MsgIDType=Standard (11-bit identifier)  MsgIdentifier=103  MsgLength=4  SignalInfo={}  IDPort=off  TimestampPort=off  ErrorPort=off  RemotePort=off  LengthPort=off  StatusPort=off  BRSPort=off  ESIPort=off  DLCPort=off  ApplyMinMax=off
      settings: SourceProductBaseCode=XP,ME,VN  DataFormat=raw data
  CAN Read1 : speedgoatlib_IO602/Legacy/CAN Read  id=1  ts=-1  channel=3  messageType=CAN  canType=CAN-FD  BusOutput=off  initValues=[602 1 -1 2 1 2 0]
      settings: SourceProductName=Simulink Real-Time: Speedgoat I/O Blockset
  While Iterator : WhileIterator  MaxIters=50  WhileBlockType=do-while
  Out1 : Outport
  wires:
  CAN Read1/1 -> While Iterator/1
  CAN Read1/2 -> CAN FD Unpack/1
  CAN FD Unpack/1 -> "Byte Packing "/1
  "Byte Packing "/1 -> Out1/1

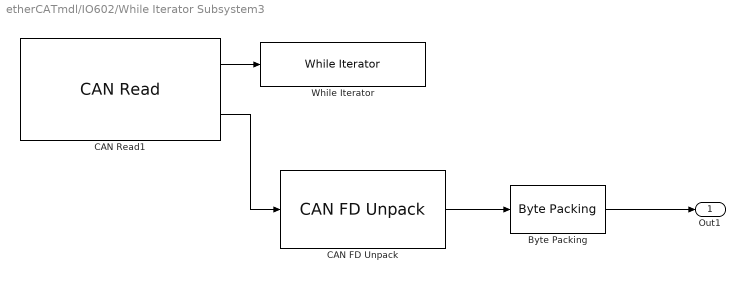
== system etherCATmdl/IO602/While Iterator Subsystem3 ==
  "Byte Packing " : slrealtimeutilitieslib/Byte Packing  MaskPackedDataType=single  MaskUnpackedDataTypes={'uint8'}  MaskAlignment=1
  CAN FD Unpack : canfdmsglib/CAN FD Unpack  MsgList=(none)  MsgName=Msg  ProtocolMode=CAN FD  MsgIDType=Standard (11-bit identifier)  MsgIdentifier=102  MsgLength=4  SignalInfo={}  IDPort=off  TimestampPort=off  ErrorPort=off  RemotePort=off  LengthPort=off  StatusPort=off  BRSPort=off  ESIPort=off  DLCPort=off  ApplyMinMax=off
      settings: SourceProductBaseCode=XP,ME,VN  DataFormat=raw data
  CAN Read1 : speedgoatlib_IO602/Legacy/CAN Read  id=1  ts=-1  channel=4  messageType=CAN  canType=CAN-FD  BusOutput=off  initValues=[602 1 -1 3 1 2 0]
      settings: SourceProductName=Simulink Real-Time: Speedgoat I/O Blockset
  While Iterator : WhileIterator  MaxIters=50  WhileBlockType=do-while
  Out1 : Outport
  wires:
  "Byte Packing "/1 -> Out1/1
  CAN FD Unpack/1 -> "Byte Packing "/1
  CAN Read1/2 -> CAN FD Unpack/1
  CAN Read1/1 -> While Iterator/1

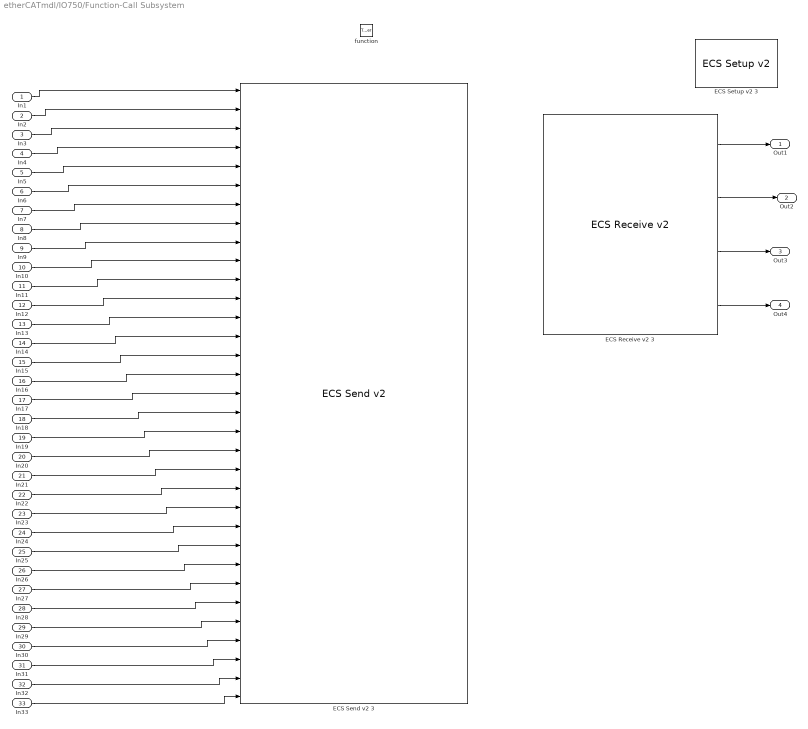
== system etherCATmdl/IO750/Function-Call Subsystem ==
  In1 : Inport
  In2 : Inport  Port=2
  In3 : Inport  Port=3
  In4 : Inport  Port=4
  In5 : Inport  Port=5
  In6 : Inport  Port=6
  In7 : Inport  Port=7
  In8 : Inport  Port=8
  In9 : Inport  Port=9
  In10 : Inport  Port=10
  In11 : Inport  Port=11
  In12 : Inport  Port=12
  In13 : Inport  Port=13
  In14 : Inport  Port=14
  In15 : Inport  Port=15
  In16 : Inport  Port=16
  In17 : Inport  Port=17
  In18 : Inport  Port=18
  In19 : Inport  Port=19
  In20 : Inport  Port=20
  In21 : Inport  Port=21
  In22 : Inport  Port=22
  In23 : Inport  Port=23
  In24 : Inport  Port=24
  In25 : Inport  Port=25
  In26 : Inport  Port=26
  In27 : Inport  Port=27
  In28 : Inport  Port=28
  In29 : Inport  Port=29
  In30 : Inport  Port=30
  In31 : Inport  Port=31
  In32 : Inport  Port=32
  In33 : Inport  Port=33
  function : TriggerPort  TriggerType=function-call  VariantControl=(inherit)
  ECS Receive v2 3 : speedgoatlib_IO750/ECS Receive v2   id=1  portType=Separate signals  sampleTime=inf  pdoTable={ 'Rx PDO1', 'myvar1', 'uint8'; 'Rx PDO1', 'myvar2', 'single'; 'Rx PDO2', 'myvar1', 'int16'; 'Rx PDO3', 'myvar1', 'double' }
      settings: SourceProductName=Simulink Real-Time: Speedgoat I/O Blockset
  ECS Send v2 3 : speedgoatlib_IO750/ECS Send v2   id=1  portType=Separate signals  sampleTime=-1  pdoTable={ 'Tx PDO1', 'myvar1', 'double'; 'Tx PDO2', 'myvar2', 'double'; 'Tx PDO3', 'myvar3', 'double'; 'Tx PDO4', 'myvar4', 'double'; 'Tx PDO5', 'myvar5', 'double'; 'Tx PDO6', 'myvar6', 'double'; 'Tx PDO7', 'myvar7', 'double'; 'Tx PDO8', 'myvar8', 'double'; 'Tx PDO9', 'myvar9', 'double'; 'Tx PDO10', 'myvar10', 'double'; 'Tx PDO11', 'myvar11', 'double'; 'Tx PDO12', 'myvar12', 'double'; 'Tx PDO13', 'myvar13', 'double'; 'Tx PDO14', 'myvar14', 'double'; 'Tx PDO15', 'myvar15', 'double'; 'Tx PDO16', 'myvar16', 'double'; 'Tx PDO17', 'myvar17', 'double'; 'Tx PDO18', 'myvar18', 'double'; 'Tx PDO19', 'myvar19', 'double'; 'Tx PDO20', 'myvar20', 'double'; 'Tx PDO21', 'myvar21', 'double'; 'Tx PDO22', 'myvar22', 'double'; 'Tx PDO23', 'myvar23', 'double'; 'Tx PDO24', 'myvar24', 'double'; 'Tx PDO25', 'myvar25', 'double'; 'Tx PDO26', 'myvar26', 'double'; 'Tx PDO27', 'myvar27', 'double'; 'Tx PDO28', 'myvar28', 'double'; 'Tx PDO29', 'myvar29', 'double'; 'Tx PDO30', 'myvar30', 'double'; 'Tx PDO31', 'myvar31', 'double'; 'Tx PDO32', 'myvar32', 'double'; 'Tx PDO32', 'myvar33', 'double' }
      settings: SourceProductName=Simulink Real-Time: Speedgoat I/O Blockset
  ECS Setup v2 3 : speedgoatlib_IO750/ECS Setup v2   id=1  drvLetter=C:  configurationMode=Warmstart  busSlot=-1  busStartup=Automatic  dcSync=on  vendorName='Speedgoat'  groupName='Automation'  typeName='IO750'  vendorID=hex2dec('00000001')  productCode=hex2dec('00000002')  revisionNo=hex2dec('00000003')  serialNo=hex2dec('00000004')  stationAlias=0  deviceIdent=0  rxPdoMapping={ 'Rx PDO1', 'myvar1', 'uint8'; 'Rx PDO1', 'myvar2', 'single'; 'Rx PDO2', 'myvar1', 'int16'; 'Rx PDO3', 'myvar1', 'double' }  rxPdoCfg=0  rxPdoNames=,Steuerwort,Steuerwort,Statuswort  rxVarNames=,AUS0,padding,AUS1  txPdoMapping={ 'Tx PDO1', 'myvar1', 'double'; 'Tx PDO2', 'myvar2', 'double'; 'Tx PDO3', 'myvar3', 'double'; 'Tx PDO4', 'myvar4', 'double'; 'Tx PDO5', 'myvar5', 'double'; 'Tx PDO6', 'myvar6', 'double'; 'Tx PDO7', 'myvar7', 'double'; 'Tx PDO8', 'myvar8', 'double'; 'Tx PDO9', 'myvar9', 'double'; 'Tx PDO10', 'myvar10', 'double'; 'Tx PDO11', 'myvar11', 'double'; 'Tx PDO12', 'myvar12', 'double'; 'Tx PDO13', 'myvar13', 'double'; 'Tx PDO14', 'myvar14', 'double'; 'Tx PDO15', 'myvar15', 'double'; 'Tx PDO16', 'myvar16', 'double'; 'Tx PDO17', 'myvar17', 'double'; 'Tx PDO18', 'myvar18', 'double'; 'Tx PDO19', 'myvar19', 'double'; 'Tx PDO20', 'myvar20', 'double'; 'Tx PDO21', 'myvar21', 'double'; 'Tx PDO22', 'myvar22', 'double'; 'Tx PDO23', 'myvar23', 'double'; 'Tx PDO24', 'myvar24', 'double'; 'Tx PDO25', 'myvar25', 'double'; 'Tx PDO26', 'myvar26', 'double'; 'Tx PDO27', 'myvar27', 'double'; 'Tx PDO28', 'myvar28', 'double'; 'Tx PDO29', 'myvar29', 'double'; 'Tx PDO30', 'myvar30', 'double'; 'Tx PDO31', 'myvar31', 'double'; 'Tx PDO32', 'myvar32', 'double'; 'Tx PDO32', 'myvar33', 'double' }  txPdoCfg=0  txPdoNames=0  txVarNames=0  sdoMapping={}  sdoCfg=0  sdoNames=0  qtyMods=[1,0,0]  moduleType=IO750  protocol=IO750  firmware=EtherCAT Slave
      settings: SourceProductName=Simulink Real-Time: Speedgoat I/O Blockset
  Out1 : Outport
  Out2 : Outport  Port=2
  Out3 : Outport  Port=3
  Out4 : Outport  Port=4
  wires:
  In33/1 -> ECS Send v2 3/33
  In14/1 -> ECS Send v2 3/14
  In15/1 -> ECS Send v2 3/15
  In9/1 -> ECS Send v2 3/9
  In11/1 -> ECS Send v2 3/11
  In13/1 -> ECS Send v2 3/13
  In12/1 -> ECS Send v2 3/12
  In10/1 -> ECS Send v2 3/10
  In4/1 -> ECS Send v2 3/4
  In5/1 -> ECS Send v2 3/5
  In6/1 -> ECS Send v2 3/6
  In7/1 -> ECS Send v2 3/7
  In17/1 -> ECS Send v2 3/17
  In3/1 -> ECS Send v2 3/3
  In16/1 -> ECS Send v2 3/16
  In19/1 -> ECS Send v2 3/19
  In31/1 -> ECS Send v2 3/31
  In22/1 -> ECS Send v2 3/22
  In8/1 -> ECS Send v2 3/8
  In28/1 -> ECS Send v2 3/28
  In29/1 -> ECS Send v2 3/29
  In23/1 -> ECS Send v2 3/23
  In27/1 -> ECS Send v2 3/27
  In2/1 -> ECS Send v2 3/2
  In30/1 -> ECS Send v2 3/30
  In24/1 -> ECS Send v2 3/24
  In21/1 -> ECS Send v2 3/21
  In32/1 -> ECS Send v2 3/32
  In18/1 -> ECS Send v2 3/18
  In25/1 -> ECS Send v2 3/25
  In26/1 -> ECS Send v2 3/26
  In20/1 -> ECS Send v2 3/20
  In1/1 -> ECS Send v2 3/1
  ECS Receive v2 3/1 -> Out1/1
  ECS Receive v2 3/2 -> Out2/1
  ECS Receive v2 3/3 -> Out3/1
  ECS Receive v2 3/4 -> Out4/1

== matlab function etherCATmdl/IO750/MATLAB Function ==
  data: nanosecondsAbs input; nanoseconds output; microseconds output; secondsIn input; miliseconds output
function [nanoseconds,microseconds,miliseconds]  = fcn(nanosecondsAbs,secondsIn)

persistent initTime
persistent seconds

if isempty(seconds)
    seconds = int32(0);
end

if isempty(initTime)|| seconds~=secondsIn
    initTime=uint64(nanosecondsAbs);
end

nanoseconds  = uint64(nanosecondsAbs-initTime);
microseconds = round(nanoseconds/1000);
miliseconds  = round(nanoseconds/1000000);


seconds=secondsIn;
